simulink model "PUSlab7sim"  (R2021b)
settings: Solver=VariableStepAuto  StartTime=0.0  StopTime=czas_systemu  MaxStep=0.1  RelTol=1e-3
values from neighbouring files (symbols this model uses):
  Cvp = cp*rop*Vp    (= 33600)    [PUSlab7.m]
  Cvw = cp*rop*Vw    (= 67200)    [PUSlab7.m]
  dqg = 0.1*q_g_N    (= 1000)    [PUSlab7.m]
  dTzew = 0    [PUSlab7.m]
  K_cp = ((a1*q_g_N)*(T_wew_N-Tp_N))/((Tp_N-T_zew_N)*(T_wew_N-T_zew_N+a1*(T_wew_N-Tp_N)))    (= 23.2558139535)    [PUSlab7.m]
  K_cw = (q_g_N)/(T_wew_N-T_zew_N+a1*(T_wew_N-Tp_N))    (= 232.558139535)    [PUSlab7.m]
  K_cwp = (a1*(q_g_N))/(T_wew_N-T_zew_N+a1*(T_wew_N-Tp_N))    (= 69.7674418605)    [PUSlab7.m]
  KpIND = KpISA    (= 3000)    [PUSlab7.m]
  L11 = [ksTwew]    [PUSlab7.m]
  L12 = [ksTp]    [PUSlab7.m]
  L21 = [kmdTwew]    [PUSlab7.m]
  L22 = [kmdTp]    [PUSlab7.m]
  M1 = [T,1]    [PUSlab7.m]
  M2 = [T_sp,1]    [PUSlab7.m]
  M3 = [T2,1]    [PUSlab7.m]
  M4 = [T3,1]    [PUSlab7.m]
  q_g_0 = q_g_N    (= 10000)    [PUSlab7.m]
  t0 = 1000    [PUSlab7.m]
  T_0_tp = 100    [PUSlab7.m]
  T_0_wew = 0    [PUSlab7.m]
  T_wew_0 = (q_g_0+K_cw*T_zew_0+a1*K_cw*Tp_0)/(K_cw+K_cwp)    [PUSlab7.m]
  T_zew_0 = T_zew_N    (= -20)    [PUSlab7.m]
  TiIND = TiISA/KpISA    (= 0.111)    [PUSlab7.m]
  To = t_2w-T2    (= 0)    [PUSlab7.m]
  To1 = t_2p-T3    (= 175)    [PUSlab7.m]
  Tp_0 = Tpzad    [PUSlab7.m]
settings Model: Creator=Mariusz  LastModifiedBy=Mariusz
settings DataIOCC: ReturnWorkspaceOutputs=off

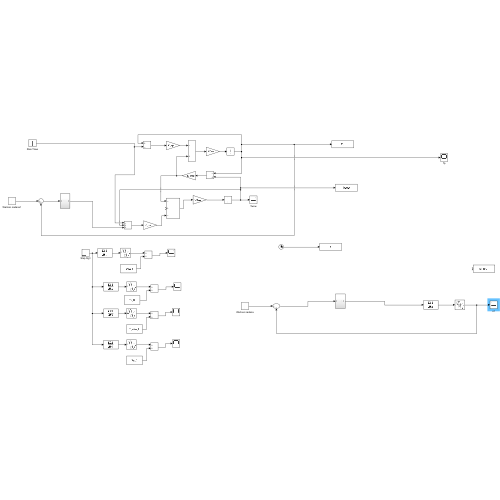
[thumbnail: Simulink's stored preview of the top-level diagram]
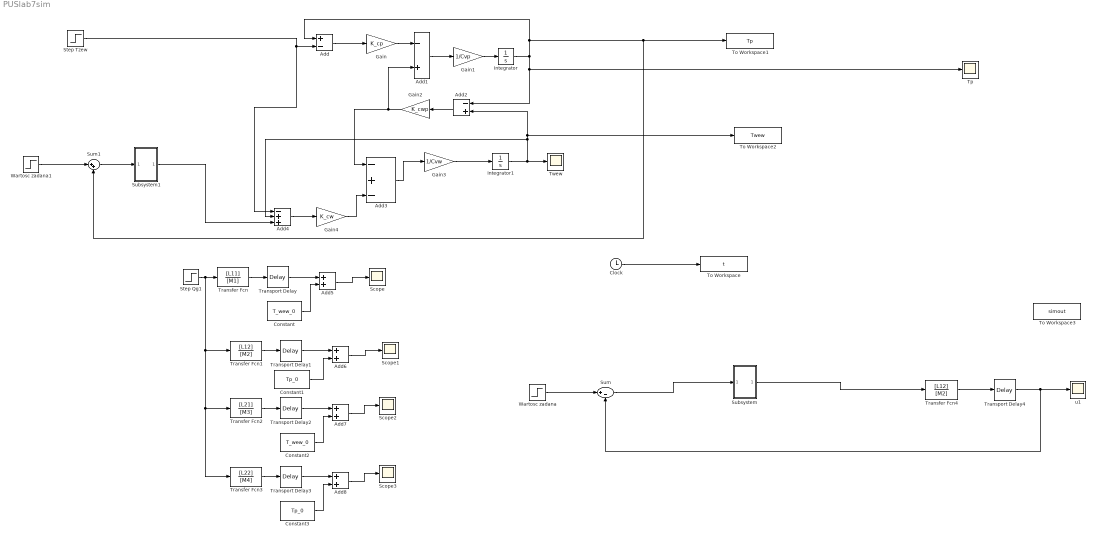
== system PUSlab7sim ==
  Add : Sum  Inputs=+-
  Add1 : Sum  Inputs=-+
  Add2 : Sum  Inputs=-+
  Add3 : Sum  Inputs=-+-
  Add4 : Sum  Inputs=-++
  Add{5..8} (4 alike) : Sum
  Clock : Clock
  Constant : Constant  Value=T_wew_0
  Constant1 : Constant  Value=Tp_0
  Constant2 : Constant  Value=T_wew_0
  Constant3 : Constant  Value=Tp_0
  Gain : Gain  Gain=K_cp
  Gain1 : Gain  Gain=1/Cvp
  Gain2 : Gain  Gain=K_cwp
  Gain3 : Gain  Gain=1/Cvw
  Gain4 : Gain  Gain=K_cw
  Integrator : Integrator  InitialCondition=Tp_0
  Integrator1 : Integrator  InitialCondition=T_wew_0
  Scope{,1..3} (4 alike) : Scope
  Step Qg1 : Step  Time=t0  After=dqg  SampleTime=0
  Step Tzew : Step  Time=t0  Before=T_zew_0  After=T_zew_0+dTzew  SampleTime=0
  Subsystem : Subsystem
  Subsystem1 : Subsystem
  Sum : Sum  Inputs=|+-
  Sum1 : Sum  Inputs=|++
  To Workspace : ToWorkspace  VariableName=t  SaveFormat=Timeseries  SampleTime=-1
  To Workspace1 : ToWorkspace  VariableName=Tp  SampleTime=-1
  To Workspace2 : ToWorkspace  VariableName=Twew  SampleTime=-1
  To Workspace3 : ToWorkspace  VariableName=simout  SaveFormat=Timeseries  SampleTime=-1
  Tp : Scope
  Transfer Fcn : TransferFcn  Numerator=[L11]  Denominator=[M1]
  Transfer Fcn1 : TransferFcn  Numerator=[L12]  Denominator=[M2]
  Transfer Fcn2 : TransferFcn  Numerator=[L21]  Denominator=[M3]
  Transfer Fcn3 : TransferFcn  Numerator=[L22]  Denominator=[M4]
  Transfer Fcn4 : TransferFcn  Numerator=[L12]  Denominator=[M2]
  Transport Delay : TransportDelay  DelayTime=T_0_wew
  Transport Delay1 : TransportDelay  DelayTime=T_0_tp
  Transport Delay2 : TransportDelay  DelayTime=To
  Transport Delay3 : TransportDelay  DelayTime=To1
  Transport Delay4 : TransportDelay  DelayTime=T_0_tp
  Twew : Scope
  Wartosc zadana : Step  Time=t0  Before=Tp_0  After=11  SampleTime=0
  Wartosc zadana1 : Step  Time=t0  Before=Tp_0  After=11  SampleTime=0
  u1 : Scope
  wires:
  Clock/1 -> To Workspace/1
  Step Tzew/1 -> Add4/1, Add/2
  Add/1 -> Gain/1
  Gain/1 -> Add1/1
  Add1/1 -> Gain1/1
  Gain1/1 -> Integrator/1
  Integrator/1 -> Add2/1, Tp/1, Sum1/2, To Workspace1/1, Add/1
  Add2/1 -> Gain2/1
  Gain2/1 -> Add3/1, Add1/2
  Integrator1/1 -> Add4/2, To Workspace2/1, Add2/2, Twew/1
  Gain3/1 -> Integrator1/1
  Add3/1 -> Gain3/1
  Gain4/1 -> Add3/3
  Add4/1 -> Gain4/1
  Transfer Fcn/1 -> Transport Delay/1
  Transport Delay/1 -> Add5/1
  Add5/1 -> Scope/1
  Constant/1 -> Add5/2
  Transport Delay1/1 -> Add6/1
  Constant1/1 -> Add6/2
  Add6/1 -> Scope1/1
  Transfer Fcn1/1 -> Transport Delay1/1
  Transport Delay2/1 -> Add7/1
  Constant2/1 -> Add7/2
  Add7/1 -> Scope2/1
  Transfer Fcn2/1 -> Transport Delay2/1
  Step Qg1/1 -> Transfer Fcn1/1, Transfer Fcn3/1, Transfer Fcn2/1, Transfer Fcn/1
  Add8/1 -> Scope3/1
  Transfer Fcn3/1 -> Transport Delay3/1
  Transport Delay3/1 -> Add8/1
  Constant3/1 -> Add8/2
  Wartosc zadana/1 -> Sum/1
  Transfer Fcn4/1 -> Transport Delay4/1
  Transport Delay4/1 -> Sum/2, u1/1
  Wartosc zadana1/1 -> Sum1/1
  Sum/1 -> Subsystem/1(In1)
  Subsystem/1(Out1) -> Transfer Fcn4/1
  Sum1/1 -> Subsystem1/1(In1)
  Subsystem1/1(Out1) -> Add4/3

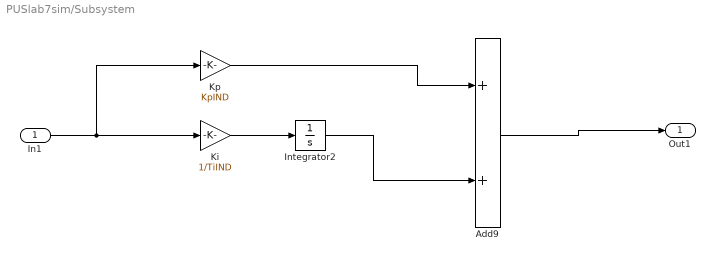
== system PUSlab7sim/Subsystem ==
  In1 : Inport
  Add9 : Sum
  Integrator2 : Integrator  InitialCondition=q_g_0
  Ki : Gain  Gain=1/TiIND
  Kp : Gain  Gain=KpIND
  Out1 : Outport
  wires:
  In1/1 -> Ki/1, Kp/1
  Integrator2/1 -> Add9/2
  Ki/1 -> Integrator2/1
  Kp/1 -> Add9/1
  Add9/1 -> Out1/1

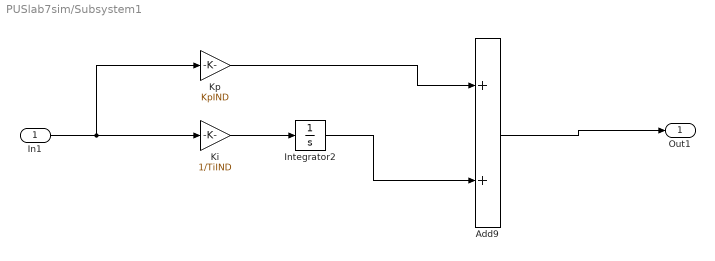
== system PUSlab7sim/Subsystem1 ==
  In1 : Inport
  Add9 : Sum
  Integrator2 : Integrator  InitialCondition=q_g_0
  Ki : Gain  Gain=1/TiIND
  Kp : Gain  Gain=KpIND
  Out1 : Outport
  wires:
  In1/1 -> Ki/1, Kp/1
  Integrator2/1 -> Add9/2
  Ki/1 -> Integrator2/1
  Kp/1 -> Add9/1
  Add9/1 -> Out1/1
